simulink model "Sensor_Complimantary_nano33"  (R2021a)
settings: Solver=FixedStepAuto  StartTime=0.0  StopTime=Inf  FixedStep=0.01  RelTol=1e-3
undefined symbols (not defined in the file or in its folder): DiscIntNeverNeededParam
libraries: arduinosensorlib x1
settings Model: SimulationMode=external  SILPILModeSetting=veronly  ExtModeTrigDuration=2  Creator=Samsung  LastModifiedBy=Samsung
settings SolverCC: AutoInsertRateTranBlk=on
settings OptimizationCC: EnhancedBackFolding=on  PassReuseOutputArgsAs=Individual arguments  ZeroExternalMemoryAtStartup=off  ZeroInternalMemoryAtStartup=off  MaxStackSize=64  OptimizeBlockOrder=speed  DifferentSizesBufferReuse=on  OptimizationCustomize=off  EfficientTunableParamExpr=on
settings DebuggingCC: ParameterTunabilityLossMsg=error
settings HardwareCC: ProdBitPerPointer=32  ProdBitPerSizeT=32  ProdBitPerPtrDiffT=32  ProdLargestAtomicInteger=Long  ProdLargestAtomicFloat=Double  ProdWordSize=32  ProdHWDeviceType=ARM Compatible->ARM Cortex
settings SFSimCC: MATLABDynamicMemAlloc=off
settings RTWCC: SystemTargetFile=ert.tlc  HardwareBoard=Arduino Nano 33 BLE Sense  TemplateMakefile=ert_default_tmf  Toolchain=Arduino ARM MBED  BuildConfiguration=Faster Runs
settings CodeAppCC: ForceParamTrailComments=on  IgnoreCustomStorageClasses=off  OperatorAnnotations=on  SimulinkDataObjDesc=on  SFDataObjDesc=on  InsertBlockDesc=on
settings ERTTargetCC: SupportContinuousTime=on  SupportVariableSizeSignals=on  ExtMode=on  ExtModeTransport=3  ExtModeStaticAlloc=on  ExtModeStaticAllocSize=65536  ExtModeMexFile=ext_xcp  ExtModeMexArgs=0 16 921600  ExtModeIntrfLevel=Level2 - Open

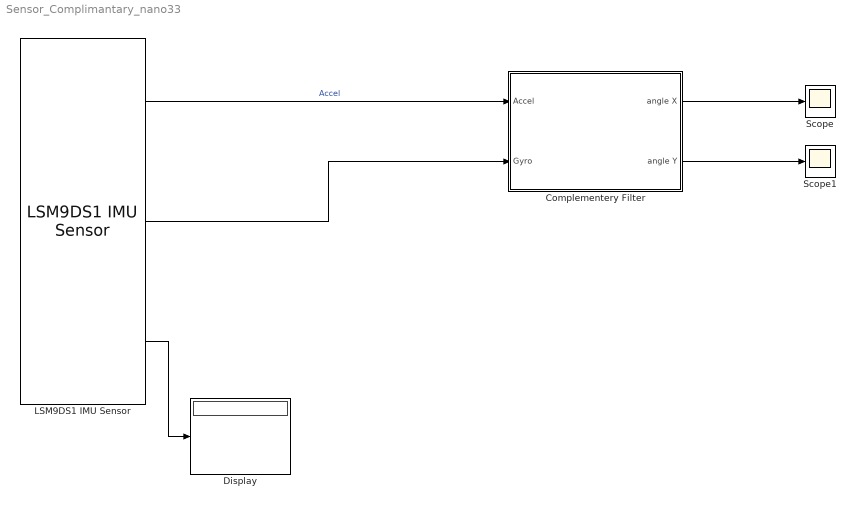
== system Sensor_Complimantary_nano33 ==
  Complementery Filter : Subsystem
  Display : Display
  LSM9DS1 IMU Sensor : arduinosensorlib/LSM9DS1 IMU Sensor  AccelandGyroAddress=0x6B  MagnetometerAddress=0x1E  EnableAccel=on  EnableGyro=on  EnableMag=on  AccelerometerOutputDataRate=119 Hz  AccelerometerFullScaleRange=+/- 16g  AccelerometerBandwidth=50 Hz  GyroscopeOutputDataRate=119 Hz  GyroscopeFullScaleRange=245 dps  GyroscopeBandwidthMode=0  GyroscopeHighPassFilterEnabled=on  GyroscopeHighPassFilterMode=0  MagnetometerOutputDataRate=40 Hz  MagnetometerFullScaleRange=+/- 4 gauss  SampleTime=0.01
      settings: SourceProductBaseCode=ARDUINO
  Scope : Scope
  Scope1 : Scope
  wires:
  LSM9DS1 IMU Sensor/3 -> Display/1
  LSM9DS1 IMU Sensor/1 -> Complementery Filter/1(Accel)  "Accel"
  LSM9DS1 IMU Sensor/2 -> Complementery Filter/2(Gyro)
  Complementery Filter/1(angle X) -> Scope/1
  Complementery Filter/2(angle Y) -> Scope1/1

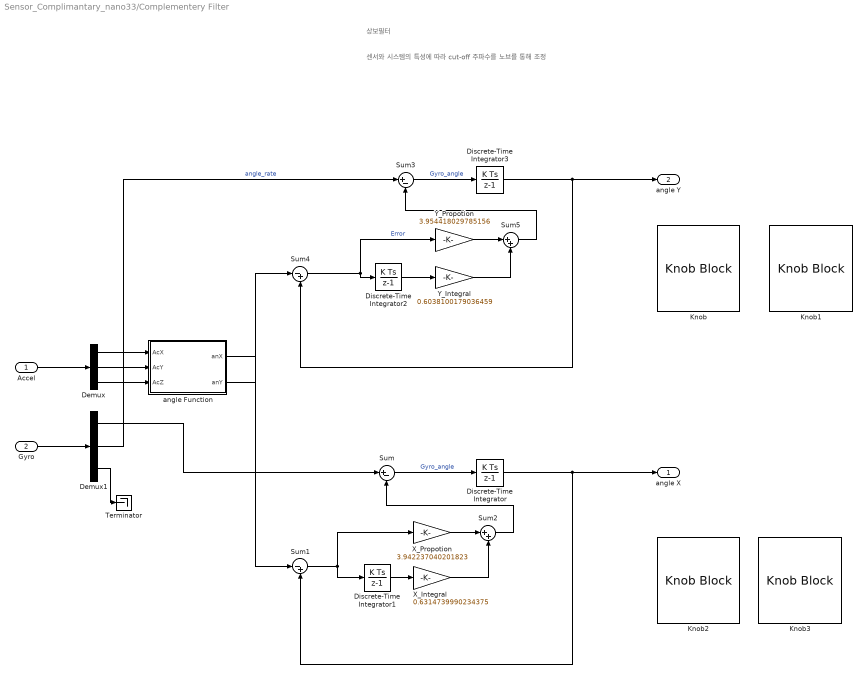
== system Sensor_Complimantary_nano33/Complementery Filter ==
  note: 센서와 시스템의 특성에 따라 cut-off 주파수를 노브를 통해 조정
  note: 상보필터
  Accel : Inport
  Gyro : Inport  Port=2
  Demux : Demux  Outputs=3
  Demux1 : Demux  Outputs=3
  Discrete-Time Integrator{,1..3} (4 alike) : DiscreteIntegrator  SampleTime=-1  ICPrevOutput=DiscIntNeverNeededParam  ICPrevScaledInput=DiscIntNeverNeededParam
  Knob : KnobBlock  ScaleMin=3  ScaleMax=4
  Knob1 : KnobBlock  ScaleMax=1
  Knob2 : KnobBlock  ScaleMin=3  ScaleMax=4
  Knob3 : KnobBlock  ScaleMax=1
  Sum : Sum  Inputs=|+-
  Sum1 : Sum  Inputs=|-+
  Sum2 : Sum  Inputs=|++
  Sum3 : Sum  Inputs=|+-
  Sum4 : Sum  Inputs=|-+
  Sum5 : Sum  Inputs=|++
  Terminator : Terminator
  X_Integral : Gain  Gain=0.6314739990234375
  X_Propotion : Gain  Gain=3.942237040201823
  Y_Integral : Gain  Gain=0.6038100179036459
  Y_Propotion : Gain  Gain=3.954418029785156
  angle Function : MATLAB Function  TreatAsAtomicUnit=on
  angle X : Outport
  angle Y : Outport  Port=2
  wires:
  X_Integral/1 -> Sum2/2
  Sum/1 -> Discrete-Time Integrator/1  "Gyro_angle"
  Discrete-Time Integrator1/1 -> X_Integral/1
  X_Propotion/1 -> Sum2/1
  Sum1/1 -> Discrete-Time Integrator1/1, X_Propotion/1
  Sum2/1 -> Sum/2
  angle Function/1(anX) -> Sum1/1
  Y_Propotion/1 -> Sum5/1
  Y_Integral/1 -> Sum5/2
  Sum3/1 -> Discrete-Time Integrator3/1  "Gyro_angle"
  Sum5/1 -> Sum3/2
  Sum4/1 -> Discrete-Time Integrator2/1, Y_Propotion/1  "Error"
  angle Function/2(anY) -> Sum4/1
  Discrete-Time Integrator3/1 -> angle Y/1, Sum4/2
  Discrete-Time Integrator/1 -> angle X/1, Sum1/2
  Demux/1 -> angle Function/1(AcX)
  Demux/2 -> angle Function/2(AcY)
  Demux/3 -> angle Function/3(AcZ)
  Accel/1 -> Demux/1
  Demux1/3 -> Terminator/1
  Gyro/1 -> Demux1/1
  Demux1/1 -> Sum/1
  Demux1/2 -> Sum3/1  "angle_rate"
  Discrete-Time Integrator2/1 -> Y_Integral/1

== matlab function Sensor_Complimantary_nano33/Complementery Filter/angle Function ==
  data: AcX input; anX output; AcY input; AcZ input; anY output
function [anX,anY] = fcn(AcX,AcY,AcZ)

anX = atan(-AcY / (sqrt(AcX^2 + AcZ^2))) * 180/pi;
anY = atan(-AcX / (sqrt(AcY^2 + AcZ^2))) * 180/pi;

end
